simulink model "LRMate200Experimentor_Robot"  (R2015b)
settings: Solver=FixedStepDiscrete  StartTime=0.0  StopTime=10.0  FixedStep=si.SolverTimeStep  RelTol=1e-3
model workspace (MATLAB code in the model file):
  | rsi = evalin('base', 'si.ri{1}');
undefined symbols (not defined in the file or in its folder): si
libraries: simulink x4
(part 2 of 2)

== system LRMate200Experimentor_Robot/ModeSelection/Basic Control Mode/SwSrc9 ==
  S0 : Constant  Value=0
  S1 : Constant
  ST1 : Outport
  ST0 : Outport  Port=2
  wires:
  S0/1 -> ST0/1
  S1/1 -> ST1/1

== system LRMate200Experimentor_Robot/ModeSelection/LTT/SwSrc13 ==
  S0 : Constant  Value=0
  S1 : Constant
  ST1 : Outport
  ST0 : Outport  Port=2
  wires:
  S0/1 -> ST0/1
  S1/1 -> ST1/1

== system LRMate200Experimentor_Robot/ModeSelection/LTT/Triggered Subsystem ==
  In1 : Inport
  Trigger : TriggerPort  PortDimensions=1
  Data Store Write : DataStoreWrite  DataStoreName=ATI_ResidueOffset
  wires:
  In1/1 -> Data Store Write/1

== system LRMate200Experimentor_Robot/ModeSelection/LTT/Triggered Subsystem1 ==
  In1 : Inport
  Trigger : TriggerPort  TriggerType=falling
  Data Store Write1 : DataStoreWrite  DialogController=Simulink.DDGSource  DataStoreName=ATI_ResidueOffset
  wires:
  In1/1 -> Data Store Write1/1

== system LRMate200Experimentor_Robot/ModeSelection/Pos Run & Jog/Triggered Subsystem2 ==
  In1 : Inport
  Trigger : TriggerPort
  Data Store Write1 : DataStoreWrite  DialogController=Simulink.DDGSource  DataStoreName=RecordPosition
  wires:
  In1/1 -> Data Store Write1/1

== system LRMate200Experimentor_Robot/ModeSelection/Pos Run & Jog/Triggered Subsystem3 ==
  In1 : Inport
  Trigger : TriggerPort  TriggerType=falling
  Data Store Write1 : DataStoreWrite  DialogController=Simulink.DDGSource  DataStoreName=RecordPosition
  wires:
  In1/1 -> Data Store Write1/1

== system LRMate200Experimentor_Robot/PLAN_INTR_FLTR/Basic/double smoothing ==
  mcmd : Inport
  1st smoothing : Subsystem
  2nd smoothing : Subsystem
  alt_efot : Outport  InitialOutput=0
  wires:
  1st smoothing/1(out_1) -> 2nd smoothing/1(in_1)
  mcmd/1 -> 1st smoothing/1(in_1)
  2nd smoothing/1(out_1) -> alt_efot/1  "MotorVelCmd[2^20rev/itp]"

== system LRMate200Experimentor_Robot/ModeSelection/Basic Control Mode/ControllerMode/SafetyOverCheck ==
  Force_limit : Constant  Value=rsi.Force_limit
  PosOverCheck : MATLAB Function  TreatAsAtomicUnit=on  SystemSampleTime=si.itp
  Rate Transition{1..5} (5 alike) : RateTransition
  SafetyTrqLimit : Constant  Value=rsi.SafetyTrqLimit
  rj_pos_limit_max : Constant  Value=rsi.rj_pos_limit_max
  rj_pos_limit_min : Constant  Value=rsi.rj_pos_limit_min
  si.BASE_Z : Constant  Value=rsi.BASE_Z
  si.RADIUS : Constant  Value=rsi.RADIUS
  si.boundary_max : Constant  Value=rsi.boundary_max
  si.boundary_min : Constant  Value=rsi.boundary_min
  si.velboundary_max : Constant  Value=rsi.velboundary_max
  SafetyOver : Outport
  wires:
  rj_pos_limit_min/1 -> PosOverCheck/9(pos_limit_min)
  Rate Transition3/1 -> PosOverCheck/6(pos_deg)
  rj_pos_limit_max/1 -> PosOverCheck/10(pos_limit_max)
  [JointPos_deg] -> Rate Transition3/1  "RBJ_pos[deg]"
  PosOverCheck/1(SafetyOver) -> SafetyOver/1
  Rate Transition1/1 -> PosOverCheck/1(TransformationM)
  si.BASE_Z/1 -> PosOverCheck/2(BASE_Z)
  si.RADIUS/1 -> PosOverCheck/3(RADIUS)
  si.boundary_min/1 -> PosOverCheck/4(boundary_min)
  si.boundary_max/1 -> PosOverCheck/5(boundary_max)
  [TransformationM] -> Rate Transition1/1
  [JointVel_degs] -> Rate Transition2/1  "JointVel [deg/s]"
  Rate Transition2/1 -> PosOverCheck/7(jvel_degsec)
  si.velboundary_max/1 -> PosOverCheck/8(velboundary_max)
  [ATI_Force] -> Rate Transition4/1
  Force_limit/1 -> PosOverCheck/12(Force_Boundary)
  Rate Transition4/1 -> PosOverCheck/11(ATI_Force)
  [MotorTrqCmd_DSA] -> Rate Transition5/1  "MotorTrqCmd [DSA]"
  Rate Transition5/1 -> PosOverCheck/13(MotorTrqCmd_DSA)
  SafetyTrqLimit/1 -> PosOverCheck/14(MotorTrqCmd_DSA_Boundary)

== system LRMate200Experimentor_Robot/ModeSelection/Basic Control Mode/ControllerMode/SetTpPrgToMemory ==
  note: Use global variable si instead of model argument rsi because block parameters are not tunable
      | with model arguments (either workspace variable or simulink parameter object, either in scalar or structure)
  Trigger : TriggerPort  TriggerType=either
  Data Store Write : DataStoreWrite  DataStoreName=DS_ExtCmd_vcmd
  Data Store Write1 : DataStoreWrite  DialogController=Simulink.DDGSource  DataStoreName=DS_ExtCmd_vcmd_EndCnt
  Data Store Write2 : DataStoreWrite  DialogController=Simulink.DDGSource  DataStoreName=DS_ExtCmd_GripperCmd
  Data Store Write8 : DataStoreWrite  DialogController=Simulink.DDGSource  DataStoreName=DS_ExtCmd_inipos
  const_ExtCmd_grippercmd : Constant  Value=si.extcmd.grippercmd  VectorParams1D=off  SampleTime=-1
  const_ExtCmd_inipos : Constant  Value=si.extcmd.inipos_t  VectorParams1D=off  SampleTime=-1
  const_ExtCmd_vcmd : Constant  Value=si.extcmd.vcmd_t  SampleTime=-1
  const_ExtCmd_vcmd_EndCnt : Constant  Value=si.extcmd.vcmd_EndCnt_t  SampleTime=-1
  wires:
  const_ExtCmd_vcmd/1 -> Data Store Write/1
  const_ExtCmd_vcmd_EndCnt/1 -> Data Store Write1/1
  const_ExtCmd_inipos/1 -> Data Store Write8/1
  const_ExtCmd_grippercmd/1 -> Data Store Write2/1

== system LRMate200Experimentor_Robot/ModeSelection/Basic Control Mode/ControllerMode/Subsystem ==
  In1 : Inport
  Bitwise Operator : simulink/Logic and Bit Operations/Bitwise Operator  logicop=AND  UseBitMask=on  BitMask=bin2dec('000000001')  BitMaskRealWorld=Stored Integer
  Bitwise Operator1 : simulink/Logic and Bit Operations/Bitwise Operator  logicop=AND  UseBitMask=on  BitMask=bin2dec('10000000')  BitMaskRealWorld=Stored Integer
  Data Type Conversion : DataTypeConversion  OutDataTypeStr=boolean
  Data Type Conversion1 : DataTypeConversion  OutDataTypeStr=boolean
  Gain : Gain  Gain=1/2^7
  Rate Transition2 : RateTransition
  Out1 : Outport
  Out2 : Outport  Port=2
  wires:
  In1/1 -> Rate Transition2/1
  Bitwise Operator/1 -> Data Type Conversion/1
  Rate Transition2/1 -> Bitwise Operator1/1, Bitwise Operator/1
  Data Type Conversion/1 -> Out1/1
  Bitwise Operator1/1 -> Gain/1
  Data Type Conversion1/1 -> Out2/1
  Gain/1 -> Data Type Conversion1/1

== system LRMate200Experimentor_Robot/PLAN_INTR_FLTR/Basic/double smoothing/1st smoothing ==
  in_1 : Inport
  1/itp : Gain  Gain=1/(si.itp*1000)  SaturateOnIntegerOverflow=on  OutDataTypeStr=Inherit: Same as input  ParamDataTypeStr=Inherit: Same as input
  Delay{2..8,21} (8 alike) : UnitDelay  SampleTime=si.tsv
  Sum : Sum  Inputs=+++++++++  SaturateOnIntegerOverflow=on  InputSameDT=on  OutDataTypeStr=Inherit: Same as first input
  Sum1 : Sum  Inputs=+-  SaturateOnIntegerOverflow=on  InputSameDT=on  OutDataTypeStr=Inherit: Same as first input
  floor3 : Rounding
  itp : Gain  Gain=si.itp*1000  SaturateOnIntegerOverflow=on  OutDataTypeStr=Inherit: Same as input  ParamDataTypeStr=Inherit: Same as input
  out_1 : Outport  InitialOutput=0
  wires:
  floor3/1 -> itp/1, out_1/1
  1/itp/1 -> floor3/1
  itp/1 -> Sum1/2
  Sum/1 -> 1/itp/1, Sum1/1
  Sum1/1 -> Delay21/1
  Delay21/1 -> Sum/9
  Delay8/1 -> Sum/8
  Delay7/1 -> Sum/7, Delay8/1
  Delay6/1 -> Sum/6, Delay7/1
  Delay5/1 -> Sum/5, Delay6/1
  Delay4/1 -> Sum/4, Delay5/1
  Delay3/1 -> Sum/3, Delay4/1
  Delay2/1 -> Sum/2, Delay3/1
  in_1/1 -> Sum/1, Delay2/1

== system LRMate200Experimentor_Robot/PLAN_INTR_FLTR/Basic/double smoothing/2nd smoothing ==
  in_1 : Inport
  1/itp : Gain  Gain=1/(si.itp*1000)  SaturateOnIntegerOverflow=on  OutDataTypeStr=Inherit: Same as input  ParamDataTypeStr=Inherit: Same as input
  Delay{2..8,21} (8 alike) : UnitDelay  SampleTime=si.tsv
  Sum : Sum  Inputs=+++++++++  SaturateOnIntegerOverflow=on  InputSameDT=on  OutDataTypeStr=Inherit: Same as first input
  Sum1 : Sum  Inputs=+-  SaturateOnIntegerOverflow=on  InputSameDT=on  OutDataTypeStr=Inherit: Same as first input
  floor3 : Rounding
  itp : Gain  Gain=si.itp*1000  SaturateOnIntegerOverflow=on  OutDataTypeStr=Inherit: Same as input  ParamDataTypeStr=Inherit: Same as input
  out_1 : Outport  InitialOutput=0
  wires:
  floor3/1 -> out_1/1, itp/1
  Sum1/1 -> Delay21/1
  itp/1 -> Sum1/2
  1/itp/1 -> floor3/1
  Sum/1 -> 1/itp/1, Sum1/1
  Delay21/1 -> Sum/9
  Delay8/1 -> Sum/8
  in_1/1 -> Sum/1, Delay2/1
  Delay2/1 -> Sum/2, Delay3/1
  Delay3/1 -> Sum/3, Delay4/1
  Delay4/1 -> Sum/4, Delay5/1
  Delay5/1 -> Sum/5, Delay6/1
  Delay6/1 -> Sum/6, Delay7/1
  Delay7/1 -> Sum/7, Delay8/1

== matlab function LRMate200Experimentor_Robot/Measurement/Tilt Angle Esimation/MATLAB Function2 ==
  data: Button input; RecordData output; DATA input
function RecordData = Panel_RecordData(Button, DATA)

persistent Button_old  

if isempty(Button_old)
    Button_old = 0;
end

RecordData = zeros(size(DATA));
if Button > Button_old                %% press the button
        RecordData = DATA;     
end
    
Button_old = Button;

== stateflow chart LRMate200Experimentor_Robot/PLAN_INTR_FLTR/Basic/INTR ==
  settings: updateMethod=DISCRETE  sampleTime=si.itp
  state Mode [parallel]
    //movetime
    settings: executionOrder=1
    state Wait
      en: cnt=0;
      fdo=0;
    state Output
      en: cnt++;
      fdo=jvel_itp;
      out_ta1=ta1;
      out_ta2=ta2;
      du: cnt++;
    state HoldOutput
      en: fdo=0;
    (default) -> Wait
    Output -> Wait [order 3] : [VRDY==0]
    HoldOutput -> Wait
    Output -> Wait [order 1] : [cnt>=movetime_itp]
    Wait -> Output : [hasChanged(PlanDone_E)]
    Output -> HoldOutput [order 2] : [hasChanged(HoldPlanDo_E)]
  state Mode1 [parallel]
    // fltr_done_E
    settings: executionOrder=2
    state Wait1
      en: cnt_fltr=0;
    state during_output
      state Output1
        en: cnt_fltr++;
        du: cnt_fltr++;
      state HoldOutput1
        en: cnt_fltr=0;
        du: cnt_fltr++;
      Output1 -> HoldOutput1 [order 2] : [hasChanged(HoldPlanDo_E)]
    (default) -> Wait1
    during_output -> Wait1 : [VRDY==0]
        | {out_ta1=0; out_ta2=0; fltr_done_E;}
    HoldOutput1 -> Wait1 : [cnt_fltr>=ta1+ta2]
        | {out_ta1=0; out_ta2=0;}
        | / fltr_done_E
    Output1 -> Wait1 [order 1] : [cnt_fltr>=movetime_itp+ta1+ta2+1]
        | {out_ta1=0; out_ta2=0;}
        | / fltr_done_E
    Wait1 -> Output1 : [hasChanged(PlanDone_E)]
  data: jvel_itp input double size=[1 6]; fdo output double size=[1 6]; cnt local double size=1; movetime_itp input double size=1; ta1 input double size=1; ta2 input double size=1; PlanDone_E input boolean size=1; out_ta1 output double size=1; out_ta2 output double size=1; HoldPlanDo_E input boolean; cnt_fltr local double; VRDY input boolean
  events: fltr_done_E output EITHER_EDGE_EVENT

== stateflow chart LRMate200Experimentor_Robot/PLAN_INTR_FLTR/Basic/FLTR ==
  settings: updateMethod=DISCRETE  sampleTime=si.itp
  (default) -> (junction 57) : {do_reset=0;
      |  do_reset2=0;}
  (junction 57) -> (junction 65) [order 2]
  (junction 57) -> (junction 60) [order 1] : [hasChanged(fltr_done_E)]
      | {do_reset=1;}
  (junction 65) -> (junction 60)
  (junction 60) -> (junction 69) [order 2]
  (junction 60) -> (junction 68) [order 1] : [hasChanged(HoldSig_E)]
      | {do_reset2=1;}
  (junction 69) -> (junction 68)
  (junction 68) -> (junction 63) : {
      | vout3  = CalVcmd_2step_x(fdo_in,fta1,fta2,6,do_reset,do_reset2,va_s);
      |        // vout3 [ deg/itp ]
      |  vout_mpls =CalRbj2Mpls(vout3,k_rbj2mpls);
      |  out_vel=vout_mpls;
      |       // out_vel [ (2^20/rev)/itp ]
      | }
  data: vin function_input double size=[1 6]; flen1a function_input double size=1; flen2a function_input double size=1; AxisNum function_input double size=1; vout2 function_output double size=[1 6]; reset function_input double; reset2 function_input double; va function_input double size=[1 6]; mf_rbj function_input double size=[1 6]; mf_k_rbj2mpls function_input double size=[6 6]; mf_mpls function_output double size=[1 6]; fdo_in input double size=[1 6]; fta1 input double size=1; fta2 input double size=1; out_vel output double size=[1 6]; fltr_done_E input boolean; do_reset local double size=1; vout3 local double size=[1 6]; k_rbj2mpls input double size=[6 6] =rsi.k_rbj2mpls; vout_mpls local double size=[1 6]; va_s input double size=[1 6]; do_reset2 local double size=1; HoldSig_E input boolean size=1
  function vout2  = CalVcmd_2step_x(vin,flen1a,flen2a,AxisNum,reset,reset2,va):
    | function vout2  = CalVcmd_2step_x(vin,flen1a,flen2a,AxisNum,reset,reset2,va)
    | %CalVcmd1 
    | %
    | %
    | %vin 
    | %flen1a: 1
    | %flen2a:  2
    | %AxisNum: )
    | %reset: 1
    | %reset2: 1va
    | %va: rese2=1
    | %
    | %
    | %vout2: 
    | 
    | 
    | %
    | persistent f1 %
    | persistent ci1 %f
    | persistent f2 %
    | persistent ci2 %f
    | 
    | 
    | flen_max=500; %
    | flen1=flen1a+1; %flenflen0=1flen=2
    | flen2=flen2a+1; %flenflen0=1flen=2
    | 
    | %----------
    | if isempty(f1)
    |    f1 = zeros(flen_max,6);
    | end
    | if isempty(ci1)
    |    ci1 = 0;
    | end
    | if isempty(f2)
    |    f2 = zeros(flen_max,6);
    | end
    | if isempty(ci2)
    |    ci2 = 0;
    | end
    | 
    | %--------0------------
    | if reset==1
    |     ci1=0;
    |     ci2=0;
    |     
    |     %-----------------------------
    |     %0
    |     f1 = zeros(flen_max,6); 
    |     f2 = zeros(flen_max,6);
    |     %------------------------------
    | 
    | end
    | 
    | %--------va---------
    | if reset2==1
    |     ci1=0;
    |     ci2=0;
    |     
    |     %-----------------------------
    |     %va
    |     f1 = [ones(flen_max,1)*va(1,1) ...
    |           ones(flen_max,1)*va(1,2) ...
    |           ones(flen_max,1)*va(1,3) ...
    |           ones(flen_max,1)*va(1,4) ...
    |           ones(flen_max,1)*va(1,5) ...
    |           ones(flen_max,1)*va(1,6)]; 
    |       
    |       
    |     f2 = f1;
    |     %------------------------------
    | 
    | end
    | 
    | %---------1--------------
    | if ci1>=flen1
    |     ci1=0;
    | end
    | ci1=ci1+1;
    | f1(ci1,:)=vin;
    | 
    | %----------------------
    | %sum
    | %
    | vout1=sum(f1(1:flen1,:),1)/flen1;
    | %----------------------
    | 
    | %---------2--------------
    | if ci2>=flen2
    |     ci2=0;
    | end
    | ci2=ci2+1;
    | f2(ci2,:)=vout1;
    | 
    | %----------------------
    | %sum
    | %
    | vout2=sum(f2(1:flen2,:),1)/flen2;
    | %----------------------
    | 
    | end
  function mf_mpls  = CalRbj2Mpls(mf_rbj,mf_k_rbj2mpls):
    | function mf_mpls  = CalRbj2Mpls(mf_rbj,mf_k_rbj2mpls)
    | %CalRbj2Mpls 
    | %
    | %
    | %mf_rbj [deg] [1X6]
    | %       6J3J2
    | %      
    | %mf_k_rbj2mpls  
    | 
    | 
    | mf_mpls=(mf_k_rbj2mpls*mf_rbj')';
    | 
    | 
    | end

== stateflow chart LRMate200Experimentor_Robot/PLAN_INTR_FLTR/Basic/PLAN ==
  (default) -> (junction 10)
  (junction 10) -> (junction 25) [order 2] : [IniState == 1]
      | { [jpos_diff,jvel_s,jvel_itp_s,movetime_itp,ta1_s,ta2_s]=CalPlan ...
      |     (jvelmax_s,AccelTime1_s,AccelTime2_s,itp_s,AxisNum_s, ...
      |      pos1,pos3); }
  (junction 10) -> (junction 25) [order 1] : [IniState == 0]
      | { [jpos_diff,jvel_s,jvel_itp_s,movetime_itp,ta1_s,ta2_s]=CalPlan ...
      |     (jvelmax_s,AccelTime1_s,AccelTime2_s,itp_s,AxisNum_s, ...
      |      pos1,pos2); }
  (junction 25) -> (junction 38) : { PlanDone_E; }
  data: jvelmax function_input double size=[1 6]; AccelTime1 function_input double size=[1 6]; AccelTime2 function_input double size=[1 6]; itp function_input double size=1; AxisNum function_input double size=1; jpos1 function_input double size=[1 6]; jpos2 function_input double size=[1 6]; Pdiff function_output double size=[1 6]; jvel function_output double size=[1 6]; jvel_itp function_output double size=[1 6]; MoveTime function_output double size=1; taconsE1 function_output double size=1; taconsE2 function_output double size=1; ta1 temporary double size=[1 6]; ta2 temporary double size=[1 6]; pos1 input double size=6; jvelmax_s input double size=6 =si.jvelmax; AccelTime1_s input double size=6 =si.AccelTime1_s; AccelTime2_s input double size=6 =si.AccelTime2_s; itp_s local double size=1 =si.itp; AxisNum_s local double size=1 =si.AxisNum; jpos_diff output double size=6; jvel_s output double size=6; jvel_itp_s output double size=6; movetime_itp output double size=1; ta1_s output double size=1; ta2_s output double size=1; pos2 input double size=[1 6]; IniState input double; pos3 input double
  events: PlanDo_E input EITHER_EDGE_EVENT; PlanDone_E output EITHER_EDGE_EVENT
  function [Pdiff,jvel,jvel_itp,MoveTime,taconsE1,taconsE2] = CalPlan ...:
    | function [Pdiff,jvel,jvel_itp,MoveTime,taconsE1,taconsE2] = CalPlan ...
    |      ( jvelmax,AccelTime1,AccelTime2,itp,AxisNum,jpos1,jpos2)
    | %CalPlan PLAN
    | % 
    | %
    | %itp: itp[s]
    | %
    | %
    | %
    | %Pdiff: 1Ax
    | %jvel: 1Ax[deg/s]
    | %jvel_itp: 1Ax[deg/itp]
    | %MoveTime: MOVE_TIME[itp]
    | %taconsE1: 1[itp]
    | %taconsE2: 2[itp]
    | 
    | 
    | %
    | Pdiff=jpos2-jpos1;
    | Pdiff_abs=abs(Pdiff);
    | 
    | ta1=ceil((AccelTime1/1000)/itp); %1[itp]
    | ta2=ceil((AccelTime2/1000)/itp); %2[itp]
    | 
    | 
    | if all(Pdiff_abs==[0 0 0 0 0 0])
    |     %
    |     
    | %     jvel=zeros(1,AxisNum);  %zerosstateFlow
    |     jvel=[0 0 0 0 0 0];
    |     jvel_itp=[0 0 0 0 0 0];
    |     MoveTime=0;
    |     taconsE1=0;
    |     taconsE2=0;
    |  
    | else
    | 
    |     %
    |     %MoveTime0[s]
    |     [MoveTime0,maxMvtime_index]=max(Pdiff_abs./jvelmax);
    |     %MoveTime[itp]
    |     MoveTime=ceil(MoveTime0/itp);
    | 
    |     %
    |     jvel_itp=Pdiff/MoveTime;
    |     jvel=jvel_itp/itp;
    | 
    |     %
    |     ta_ratio=abs(jvel)./jvelmax;
    |     tacons1G=ceil(ta1.*ta_ratio);
    |     tacons2G=ceil(ta2.*ta_ratio);
    | 
    |     %
    |     [maxtacons,maxta_index]=max(tacons1G+tacons2G);
    |     taconsE1=tacons1G(maxta_index);
    |     taconsE2=tacons2G(maxta_index);
    |         %tacons1,tacons2ta_ratio
    |         %ta_ratio
    | end
    | 
    | end

== stateflow chart LRMate200Experimentor_Robot/PLAN_INTR_FLTR/JOG C/JOGC ==
  settings: updateMethod=DISCRETE  sampleTime=si.itp
  state Wait
    en: fdo=0;
  state Output_state
    state Output
      en:  fdo =JogC_CartesianVel(jog_axis_no,jog_speed_ratio,jog_direction);
      du:  fdo =JogC_CartesianVel(jog_axis_no,jog_speed_ratio,jog_direction);
    state HoldOutput
      en: fdo=0;
      cnt_fltr=0;
      du: cnt_fltr++;
    Output -> HoldOutput : [hasChanged(JogCCmd_E)]
  (default) -> Wait
  Output_state -> Wait : [VRDY==0]
      | / fltr_done_E_C
  (junction 114) -> Wait
  Wait -> Output : [hasChanged(JogCCmd_E)]
  HoldOutput -> (junction 114) : [cnt_fltr>=50]
      | / fltr_done_E_C
  data: jog_axis_no_in function_input double size=1; vel function_output double size=[1 6]; jog_speed_ratio_in function_input double size=1; jog_direction_in function_input double size=1; fdo output double size=[1 6]; cnt_fltr local double; VRDY input boolean; JogCCmd_E input boolean; jog_axis_no input double; jog_speed_ratio input double; jog_direction input double
  events: fltr_done_E_C output EITHER_EDGE_EVENT
  function vel  = JogC_CartesianVel(jog_axis_no_in,jog_speed_ratio_in,jog_direction_in):
    | function vel  = JogC_CartesianVel(jog_axis_no_in,jog_speed_ratio_in,jog_direction_in)
    | 
    | % Maximum Vel
    | Vmax = [0.1, 0.1, 0.1, 0.1745, 0.1745, 0.1745] ;    %   m/s         % rad/s
    | 
    | % Tool frame Velcoticy in Cartesian Space
    | vel = zeros(1,6);
    | vel(jog_axis_no_in)=Vmax(jog_axis_no_in)*(jog_speed_ratio_in/100)*jog_direction_in; %
    | 
    | end

== stateflow chart LRMate200Experimentor_Robot/PLAN_INTR_FLTR/Basic/Switch_VelCmdSource (MATLABchart) ==
  state ext_vel1
    en: cnt_itp=1;
    out_VelCmd=jogC_VelCmd';
    du: cnt_itp=cnt_itp+1;
    out_VelCmd= jogC_VelCmd';
  state ext_vel2
    en: cnt_itp=1;
    out_VelCmd=Force_VelCmd';
    du: cnt_itp=cnt_itp+1;
    out_VelCmd= Force_VelCmd';
  note: ext_vel(cnt_itp,:)
      | MATLAB
  state ini00_wait
  state ext_vel3
    en: cnt_itp=1;
    out_VelCmd=LTT_VelCmd';
    du: cnt_itp=cnt_itp+1;
    out_VelCmd= LTT_VelCmd';
  state inner_vel
    en: out_VelCmd=inner_VelCmd';
    du: out_VelCmd=inner_VelCmd';
  state ext_vel4
    en: cnt_itp=1;
    out_VelCmd=TI_VelCmd';
    du: cnt_itp=cnt_itp+1;
    out_VelCmd= TI_VelCmd';
  state ext_vel
    en: cnt_itp=1;
    out_VelCmd= ext_VelCmd';
    du: cnt_itp=cnt_itp+1;
    out_VelCmd= ext_VelCmd';
    %  ext_vel(cnt_itp,:)
    %  MATLAB
  state ext_vel_hold
    en: out_VelCmd=inner_VelCmd';
    du: out_VelCmd=inner_VelCmd';
  inner_vel -> ext_vel1 [order 5] : [hasChanged(JogCCmd_E)]
  (default) -> ini00_wait
  ext_vel1 -> inner_vel : [hasChanged(fltr_done_E_C)]
  inner_vel -> ext_vel2 [order 2] : [hasChanged(ForceCmd_E)]
  ext_vel2 -> inner_vel : [hasChanged(fltr_done_E_F)]
  ini00_wait -> inner_vel
  inner_vel -> ext_vel3 [order 4] : [hasChanged(LTTCmd_E)]
  ext_vel_hold -> inner_vel : [hasChanged(fltr_done_E)]
  ext_vel3 -> inner_vel : [hasChanged(fltr_done_E_L)]
  ext_vel -> inner_vel [order 2] : [hasChanged(fltr_done_E)]
  inner_vel -> ext_vel [order 1] : [hasChanged(ExtCmd_E)]
  ext_vel4 -> inner_vel : [hasChanged(fltr_done_E_TI)]
  inner_vel -> ext_vel4 [order 3] : [hasChanged(TICmd_E)]
  ext_vel -> ext_vel_hold [order 1] : [hasChanged(ExtCmd_Hold_E)]
  data: inner_VelCmd input double size=[1 6]; out_VelCmd output double size=6; cnt_itp local; ext_VelCmd input; ExtCmd_Hold_E input boolean size=1; fltr_done_E input boolean size=1; ExtCmd_E input boolean size=1; fltr_done_E_C input; JogCCmd_E input; jogC_VelCmd input; Force_VelCmd input; ForceCmd_E input; fltr_done_E_F input; fltr_done_E_L input; LTT_VelCmd input; LTTCmd_E input; fltr_done_E_TI input; TI_VelCmd input; TICmd_E input

== stateflow chart LRMate200Experimentor_Robot/PLAN_INTR_FLTR/Basic/FDO Source SW ==
  state CmdMode [parallel]
    settings: executionOrder=1
    state InnerCmd
      en,du:
      out_fdo=in1_fdo;
      out_ta1=in1_ta1;
      out_ta2=in1_ta2;
    state ReadyForCmd
      en:
      out_fdo=zero_fdo;
      out_ta1=0;
      out_ta2=0;
    state ExtCmd
      en,du:
      out_fdo=in2_fdo;
      out_ta1=in2_ta1;
      out_ta2=in2_ta2;
    state JogCmd
      en,du:
      out_fdo=in3_fdo;
      out_ta1=in3_ta1;
      out_ta2=in3_ta2;
    (default) -> (junction 76)
    (junction 74) -> (junction 76)
    (junction 76) -> ReadyForCmd
    (junction 65) -> (junction 74)
    ReadyForCmd -> InnerCmd [order 1] : [hasChanged(InnerCmd_E)]
    InnerCmd -> (junction 65) : fltr_done_E
    (junction 66) -> (junction 65)
    ReadyForCmd -> ExtCmd [order 2] : [hasChanged(ExtCmd_E)]
    ReadyForCmd -> JogCmd [order 3] : [hasChanged(JogCmd_E)]
    ExtCmd -> (junction 66) : fltr_done_E
    (junction 69) -> (junction 66)
    JogCmd -> (junction 69) : fltr_done_E
  state fltr_done_E_State [parallel]
    settings: executionOrder=2
    state fltr_done_E_Check
    (default) -> fltr_done_E_Check
    fltr_done_E_Check -> fltr_done_E_Check : [hasChanged(in1_fltr_done_E) |  hasChanged(in2_fltr_done_E) | hasChanged(in3_fltr_done_E)]
        | {out_fltr_done_E; }
        | / send(fltr_done_E,CmdMode);
  data: out_fdo output double size=[1 6]; out_ta1 output double; out_ta2 output double; in1_fdo input double size=[1 6]; in1_ta1 input double size=1; in1_ta2 input double size=1; in1_fltr_done_E input boolean; in2_fdo input double size=[1 6]; in2_ta1 input double size=1; in2_ta2 input double size=1; in2_fltr_done_E input boolean; in3_fdo input double size=[1 6]; in3_ta1 input double size=1; in3_ta2 input double size=1; in3_fltr_done_E input boolean; InnerCmd_E input boolean size=1; ExtCmd_E input boolean size=1; JogCmd_E input boolean size=1; zero_fdo constant double size=[1 6] =[0 0 0 0 0 0]
  events: out_fltr_done_E output EITHER_EDGE_EVENT; fltr_done_E local FUNCTION_CALL_EVENT

== stateflow chart LRMate200Experimentor_Robot/PLAN_INTR_FLTR/Basic/extcmd ==
  state ini00_wait
  state during_output
    state ext_vel
      en:
      out_VelCmd= DS_ExtCmd_vcmd(cnt_itp,:);
      out_GripperCmd= DS_ExtCmd_GripperCmd(cnt_itp,:);
      du:
      cnt_itp=cnt_itp+1;
      out_VelCmd= DS_ExtCmd_vcmd(cnt_itp,:);
      out_GripperCmd= DS_ExtCmd_GripperCmd(cnt_itp,:);
    state HoldDo
      en:
      out_vel_at_hold=out_VelCmd;
      out_VelCmd=[0 0 0 0 0 0];
      out_GripperCmd=[0 0 0 0 0 0];
      cnt_hold=0;
      du:
      cnt_hold = cnt_hold + 1;
    ext_vel -> HoldDo [order 1] : [hasChanged(ExtCmd_Hold_E)]
  (default) -> ini00_wait
  during_output -> ini00_wait : [VRDY==0]
      | {out_VelCmd=[0 0 0 0 0 0];
      | out_GripperCmd=[0 0 0 0 0 0];
      | fltr_done_E;}
  HoldDo -> ini00_wait : [cnt_hold>=hold_ta1+hold_ta2]
      | {fltr_done_E;}
  ext_vel -> ini00_wait [order 2] : [cnt_itp>= DS_ExtCmd_vcmd_EndCnt]
      | {out_VelCmd=[0 0 0 0 0 0];
      | out_GripperCmd=[0 0 0 0 0 0];
      | fltr_done_E;}
  ini00_wait -> ext_vel : [hasChanged(ExtCmd_E)]
      | {cnt_itp=1;}
  data: ExtCmd_E input boolean size=1; out_VelCmd output double size=[1 6]; cnt_itp local; DS_ExtCmd_vcmd data_store_memory; DS_ExtCmd_vcmd_EndCnt data_store_memory; ExtCmd_Hold_E input boolean size=1; out_vel_at_hold output size=[1 6]; hold_ta1 input; hold_ta2 input; cnt_hold local; VRDY input boolean; DS_ExtCmd_GripperCmd data_store_memory; out_GripperCmd output double size=[1 6]
  events: fltr_done_E output EITHER_EDGE_EVENT

== matlab function LRMate200Experimentor_Robot/Measurement/Force Sensor/Gravity Compensator ==
  data: W output; T input; PayloadG input; PayloadCG input
function W = gcomp(T,PayloadG,PayloadCG)
%#Gravity Compensation
R = T(1:3,1:3,6);   % Use the tool frame (J6 frame), which is the same as ATI frame
Fg = R'*PayloadG;
Tg = cross(PayloadCG,Fg);
W = [Fg; Tg];

== stateflow chart LRMate200Experimentor_Robot/PLAN_INTR_FLTR/JOG C/JOG1 ==
  settings: updateMethod=DISCRETE  sampleTime=si.itp
  state Wait
    en: fdo=0;
  state Output_state
    state Output
      en: [fdo,out_ta1,out_ta2] = CalJogAccTime ...
      (jog_jvelmax_s,AccelTime1_s,AccelTime2_s,itp_s, ...
      jog_axis_no_s,jog_speed_ratio_s,jog_direction_s);
    state HoldOutput
      en: fdo=0;
      cnt_fltr=0;
      du: cnt_fltr++;
    Output -> HoldOutput : [hasChanged(JogCCmd_E)]
  (default) -> Wait
  Output_state -> Wait : [VRDY==0]
      | {out_ta1=0; out_ta2=0;}
      | / fltr_done_E_C
  (junction 114) -> Wait
  Wait -> Output : [hasChanged(JogCCmd_E)]
  HoldOutput -> (junction 114) : [cnt_fltr>=out_ta1+out_ta2]
      | {out_ta1=0; out_ta2=0;}
      | / fltr_done_E_C
  data: jog_jvelmax function_input double size=[1 6]; AccelTime1 function_input double size=[1 6]; AccelTime2 function_input double size=[1 6]; itp function_input double size=1; jog_axis_no function_input double size=1; jvel_itp_vec function_output double size=[1 6]; ta1x function_output double size=1; ta2x function_output double size=1; ta1 temporary double size=1; ta2 temporary double size=1; jog_speed_ratio function_input double size=1; jog_direction function_input double size=1; fdo output double size=[1 6]; out_ta1 output double size=1; out_ta2 output double size=1; cnt_fltr local double; AccelTime1_s local double size=[1 6] =si.jog_AccelTime1_s; AccelTime2_s local double size=[1 6] =si.jog_AccelTime2_s; itp_s local double =si.itp; jog_jvelmax_s local double size=[1 6] =si.jog_jvelmax; jog_axis_no_s input double size=1; jog_speed_ratio_s input double size=1; jog_direction_s input double size=1; VRDY input boolean; JogCCmd_E input boolean
  events: fltr_done_E_C output EITHER_EDGE_EVENT
  function [jvel_itp_vec,ta1x,ta2x] = CalJogAccTime ...:
    | function [jvel_itp_vec,ta1x,ta2x] = CalJogAccTime ...
    |      (jog_jvelmax,AccelTime1,AccelTime2,itp,jog_axis_no,jog_speed_ratio,jog_direction)
    | %CalJogAccTime JOGFDO
    | % 
    | %
    | %jog_jvelmax: JOG[deg/s] 1Ax
    | %AccelTime1: JOG1[ms] 1Ax
    | %AccelTime2: JOG2[ms] 1Ax
    | %itp: itp[s]
    | %jog_axis_no: JOG(:16)
    | %jog_speed_ratio: JOG[%]
    | %jog_direction:JOG -1,0,1
    | %
    | %jvel_itp_vec: 1Ax[deg/itp]
    | %ta1x: 1[itp]
    | %ta2x: 2[itp]
    | 
    | ta1=ceil((AccelTime1(jog_axis_no)/1000)/itp); %1[itp] 
    | ta2=ceil((AccelTime2(jog_axis_no)/1000)/itp); %2[itp] 
    |     
    | %jog1itp[deg/itp]
    | jvel_itp_max=jog_jvelmax(jog_axis_no)*itp; %
    | %JOG[deg/itp]
    | jvel_itp=jvel_itp_max*(jog_speed_ratio/100)*jog_direction; %
    | 
    | %
    | jvel_itp_vec=zeros(1,6); %
    | jvel_itp_vec(jog_axis_no)=jvel_itp; %
    | 
    | %JOG
    | ta_ratio=abs(jvel_itp)/jvel_itp_max;
    | ta1x=ceil(ta1*ta_ratio);
    | ta2x=ceil(ta2*ta_ratio);
    | 
    | end

== stateflow chart LRMate200Experimentor_Robot/PLAN_INTR_FLTR/Basic/JOG ==
  settings: updateMethod=DISCRETE  sampleTime=si.itp
  state Wait
    en: fdo=0;
  state Output_state
    state Output
      en: [fdo,out_ta1,out_ta2] = CalJogAccTime ...
      (jog_jvelmax_s,AccelTime1_s,AccelTime2_s,itp_s, ...
      jog_axis_no_s,jog_speed_ratio_s,jog_direction_s);
    state HoldOutput
      en: fdo=0;
      cnt_fltr=0;
      du: cnt_fltr++;
    Output -> HoldOutput : [hasChanged(JogCmd_E)]
  (default) -> Wait
  Output_state -> Wait : [VRDY==0]
      | {out_ta1=0; out_ta2=0;}
      | / fltr_done_E
  (junction 114) -> Wait
  Wait -> Output : [hasChanged(JogCmd_E)]
  HoldOutput -> (junction 114) : [cnt_fltr>=out_ta1+out_ta2]
      | {out_ta1=0; out_ta2=0;}
      | / fltr_done_E
  data: jog_jvelmax function_input double size=[1 6]; AccelTime1 function_input double size=[1 6]; AccelTime2 function_input double size=[1 6]; itp function_input double size=1; jog_axis_no function_input double size=1; jvel_itp_vec function_output double size=[1 6]; ta1x function_output double size=1; ta2x function_output double size=1; ta1 temporary double size=1; ta2 temporary double size=1; jog_speed_ratio function_input double size=1; jog_direction function_input double size=1; fdo output double size=[1 6]; out_ta1 output double size=1; out_ta2 output double size=1; JogCmd_E input boolean; cnt_fltr local double; AccelTime1_s input double size=[1 6] =si.jog_AccelTime1_s; AccelTime2_s input double size=[1 6] =si.jog_AccelTime2_s; itp_s local double =si.itp; jog_jvelmax_s input double size=[1 6] =si.jog_jvelmax; jog_axis_no_s input double size=1; jog_speed_ratio_s input double size=1; jog_direction_s input double size=1; VRDY input boolean
  events: fltr_done_E output EITHER_EDGE_EVENT
  function [jvel_itp_vec,ta1x,ta2x] = CalJogAccTime ...:
    | function [jvel_itp_vec,ta1x,ta2x] = CalJogAccTime ...
    |      (jog_jvelmax,AccelTime1,AccelTime2,itp,jog_axis_no,jog_speed_ratio,jog_direction)
    | %CalJogAccTime JOGFDO
    | % 
    | %
    | %jog_jvelmax: JOG[deg/s] 1Ax
    | %AccelTime1: JOG1[ms] 1Ax
    | %AccelTime2: JOG2[ms] 1Ax
    | %itp: itp[s]
    | %jog_axis_no: JOG(:16)
    | %jog_speed_ratio: JOG[%]
    | %jog_direction:JOG -1,0,1
    | %
    | %jvel_itp_vec: 1Ax[deg/itp]
    | %ta1x: 1[itp]
    | %ta2x: 2[itp]
    | 
    | ta1=ceil((AccelTime1(jog_axis_no)/1000)/itp); %1[itp] 
    | ta2=ceil((AccelTime2(jog_axis_no)/1000)/itp); %2[itp] 
    |     
    | %jog1itp[deg/itp]
    | jvel_itp_max=jog_jvelmax(jog_axis_no)*itp; %
    | %JOG[deg/itp]
    | jvel_itp=jvel_itp_max*(jog_speed_ratio/100)*jog_direction; %
    | 
    | %
    | jvel_itp_vec=zeros(1,6); %
    | jvel_itp_vec(jog_axis_no)=jvel_itp; %
    | 
    | %JOG
    | ta_ratio=abs(jvel_itp)/jvel_itp_max;
    | ta1x=ceil(ta1*ta_ratio);
    | ta2x=ceil(ta2*ta_ratio);
    | 
    | end

== matlab function LRMate200Experimentor_Robot/PLAN_INTR_FLTR/Peg Hole Insertion/MATLAB Function ==
  data: VRDY input; ForceCmd_E input; JacobianT input; TCP_Force input; TCP_Pos input; Tilt_Angle input; JointVelCmd output; CartesianVelCmd output; fltr_done_E_F output; GMRpar_Priors input; GMRpar_Mu input; GMRpar_Sigma input; GMRpar_inv_SigmaIn input; GMRpar_det_SigmaIn input
function [JointVelCmd,CartesianVelCmd,fltr_done_E_F] = ForceControl_GMR(VRDY,ForceCmd_E,JacobianT,TCP_Force, TCP_Pos,Tilt_Angle, GMRpar_Priors ,GMRpar_Mu, GMRpar_Sigma, GMRpar_inv_SigmaIn,GMRpar_det_SigmaIn)

persistent fltr_done_E_F_old timeindex ForceCme_E_open

if isempty(fltr_done_E_F_old)
    fltr_done_E_F_old = false;
    timeindex = 0;
    ForceCme_E_open = false;
end

fltr_done_E_F = false;
JointVelCmd = zeros(1,6);
CartesianVelCmd = zeros(1,6);

if VRDY == 0     % system false
    fltr_done_E_F = ~fltr_done_E_F_old;
    JointVelCmd = zeros(1,6);
    ForceCme_E_open = false;
else     % VRDY == 1 system normal
    if ForceCmd_E == 1;        % turn on Force Control
        [JointVelCmd,CartesianVelCmd] = GMR_Force2qdot(JacobianT,TCP_Force, TCP_Pos, ForceCme_E_open ,Tilt_Angle, GMRpar_Priors ,GMRpar_Mu, GMRpar_Sigma, GMRpar_inv_SigmaIn,GMRpar_det_SigmaIn);
        ForceCme_E_open = true;
        %JointVelCmd = zeros(1,6);  
        
    else %ForceCmd_E == 0;   turn off Force Control
        JointVelCmd = zeros(1,6);
        if ForceCme_E_open == true;    % only if the Force Control has even been opened, then timestep begin to increase
            timeindex = timeindex + 1;
        end
        if timeindex > 50            % 50 timestep for smooth stop when Force Control turned off
            fltr_done_E_F = ~fltr_done_E_F_old;
            timeindex = 0 ;
            ForceCme_E_open = false;
        end
    end
end

%JointVelCmd = zeros(1,6);        %%% !!!!!!!!!!!!!!!

fltr_done_E_F_old = fltr_done_E_F;

== matlab function LRMate200Experimentor_Robot/PLAN_INTR_FLTR/JOG C/MATLAB Function1 ==
  data: Jacobian input; qdot output; vel input
function qdot = vel2qdot(Jacobian, vel)

q_dot = Jacobian\(vel');
qdot = q_dot';

== matlab function LRMate200Experimentor_Robot/PLAN_INTR_FLTR/LTT/MATLAB Function2 ==
  data: VRDY input; JointVelCmd output; LTTCmd_E input; LTT_ButtonE input; Jacobian input; LTT_Force input; fltr_done_E_L output; LTT_Gain input; LTT_Speed_Limit input
function [JointVelCmd, fltr_done_E_L] = ForceControl_LTT(VRDY, LTTCmd_E, LTT_ButtonE, Jacobian, LTT_Force, LTT_Gain, LTT_Speed_Limit)

persistent fltr_done_E_L_old

if isempty(fltr_done_E_L_old)
    fltr_done_E_L_old = false;
end

fltr_done_E_L = false;
JointVelCmd = zeros(1,6);

if VRDY == 0     % system false
    fltr_done_E_L = ~fltr_done_E_L_old;
    JointVelCmd = zeros(1,6); 
else     % VRDY == 1 system normal
    if (LTTCmd_E == 1) && (LTT_ButtonE == true) ;    % turn on Lead Through Teaching
        JointVelCmd = LTT_Force2qdot(Jacobian, LTT_Force, LTT_Gain, LTT_Speed_Limit);       
    elseif LTTCmd_E == 0            %LTTCmd_E == 0;   turn off Lead Through Teaching
        JointVelCmd = zeros(1,6);
        fltr_done_E_L = ~fltr_done_E_L_old;
    else
        JointVelCmd = zeros(1,6);
    end
end

fltr_done_E_L_old = fltr_done_E_L;

== matlab function LRMate200Experimentor_Robot/Measurement/LTT Handle/MATLAB Function ==
  data: LTT_Button input; LTTCmd_E input; RecordData output; DATA input; clock input; LTT_ButtonEnable output; RecordDataOn input; Record_Flag_Other input; Record_Flag_Self output
function [RecordData,  LTT_ButtonEnable, Record_Flag_Self] = LTT_RecordData(LTT_Button, LTTCmd_E, DATA, clock, RecordDataOn, Record_Flag_Other)

persistent LTT_Button_old  clock_click  GripperCmd_old

if isempty(LTT_Button_old)
    LTT_Button_old = 0;
    clock_click = 0;
    GripperCmd_old = zeros(6,1);
end

RecordData = zeros(size(DATA));

Record_Flag_Self = false;

if (RecordDataOn || Record_Flag_Other) && (clock - clock_click > 0.5)
    % (RecordDataOn used for Host PC controlled action). Do not record
    % data again within 0.5 sec (when RecordDataOn is reset)
    RecordData = DATA;
    %Record_Flag_Self = true;
    clock_click = clock;
end

if ~isequal(DATA(end-11:end-6), GripperCmd_old)    % if GripperCmd changes, also record data
    if clock > 2,  RecordData = DATA;  Record_Flag_Self = true;  end      % Record after application starts for 2 secs (initialization time)
    GripperCmd_old = DATA(end-11:end-6);
end

if LTTCmd_E     % LTT mode is enabled
    if LTT_Button > LTT_Button_old                  % press the button
        if (clock - clock_click < 1) && (clock - clock_click > 0.1)     % if double click, record data
            RecordData = DATA;
            Record_Flag_Self = true;
        end
        clock_click = clock;
    end
else
    GripperCmd_old = DATA(end-11:end-6);
end

LTT_ButtonEnable = false;
if LTT_Button == 1 && (clock - clock_click > 1)
    LTT_ButtonEnable = true;
end

LTT_Button_old = LTT_Button;

== matlab function LRMate200Experimentor_Robot/Measurement/Force Sensor/MATLAB Function6 ==
  data: ATI_Force input; TCP_Force output; L_ATI2TCP input; LTT_Force output; L_ATI2LTT input
function [TCP_Force, LTT_Force] = ForceTransform(ATI_Force, L_ATI2TCP, L_ATI2LTT)

% Add L_ATI2TCP and L_ATI2LTT as additional inputs and LTT_Force as additional output.
% -- Wenjie Chen, 2016/06/23

% ATI_Force: force/torque values at ATI sensor origin and sensor frame
% TCP_Force: force/torque values at TCP origin and robot tool frame
% LTT_Force: force/torque values at LTT handle grasping point and robot tool frame

% ATI frame and Tool frame have the same XYZ directions
TCP_Force = ATI_Force;
TCP_Force(4) = ATI_Force(4) + ATI_Force(2)*L_ATI2TCP(3) - ATI_Force(3)*L_ATI2TCP(2);
TCP_Force(5) = ATI_Force(5) - ATI_Force(1)*L_ATI2TCP(3) + ATI_Force(3)*L_ATI2TCP(1);
TCP_Force(6) = ATI_Force(6) + ATI_Force(1)*L_ATI2TCP(2) - ATI_Force(2)*L_ATI2TCP(1);

% ATI frame and Tool frame have the same XYZ directions
LTT_Force = ATI_Force;
LTT_Force(4) = ATI_Force(4) + ATI_Force(2)*L_ATI2LTT(3) - ATI_Force(3)*L_ATI2LTT(2);
LTT_Force(5) = ATI_Force(5) - ATI_Force(1)*L_ATI2LTT(3) + ATI_Force(3)*L_ATI2LTT(1);
LTT_Force(6) = ATI_Force(6) + ATI_Force(1)*L_ATI2LTT(2) - ATI_Force(2)*L_ATI2LTT(1);

== matlab function LRMate200Experimentor_Robot/Device Control/Gripper Input/MATLAB Function ==
  data: Green_Button input; Gripper_Mode output; Gripper_Drive output; clock input; Desired_Mode input
% Wenjie Chen, FANUC Corporation, 2016/06/29
% To control the gripper action by buttons. Here only two gripper modes are
% considered: 0-fully open and Desired_Mode. When double click the green
% button, the gripper mode is changed and executed.

function [Gripper_Mode, Gripper_Drive] = Gripper_Action(Green_Button, clock, Desired_Mode)

persistent Green_Button_old  Gripper_Mode_old  Gripper_Drive_old  clock_click

if isempty(Green_Button_old)
    Green_Button_old = 0;
    Gripper_Mode_old = 0;
    Gripper_Drive_old = false;
    clock_click = 0;
end

Gripper_Mode = Gripper_Mode_old;
if Gripper_Drive_old && (clock - clock_click < 0.032)   % if it is driving, make sure it should last at least 30ms
    Gripper_Drive = Gripper_Drive_old;
else
    Gripper_Drive = false;
end

if Green_Button ~= Green_Button_old                %% press the button
    if (clock - clock_click < 1) && (clock - clock_click > 0.1)      %% double click
        if Gripper_Mode_old
            Gripper_Mode = 0;
        else
            Gripper_Mode = Desired_Mode;
        end
        Gripper_Drive = true;
    end
    clock_click = clock;
end

Green_Button_old = Green_Button;
Gripper_Mode_old = Gripper_Mode;
Gripper_Drive_old = Gripper_Drive;

== matlab function LRMate200Experimentor_Robot/PLAN_INTR_FLTR/JOG C/MATLAB Function2 ==
  data: jogC_vel_cmd input; vel_cmd_C output; cur_tcp_pos input; boundary_min input; boundary_max input; Transformation_M input; T_B2W input
function vel_cmd_C = velC_cmd_adjust(jogC_vel_cmd, cur_tcp_pos, boundary_min, boundary_max, Transformation_M, T_B2W)

Rot_T2W = T_B2W(1:3,1:3) * Transformation_M(1:3,1:3,7);
vel_cmd_C_trans = Rot_T2W * jogC_vel_cmd(1:3);
slow_ratio = 0.3;
stop_zone = 0.01;
slow_zone = 0.05;

idx_out_limit = (cur_tcp_pos <= boundary_min + stop_zone * ones(3,1)) & vel_cmd_C_trans(1:3) < 0;
vel_cmd_C_trans(idx_out_limit) = 0;

idx_out_limit = (cur_tcp_pos >= boundary_max - stop_zone * ones(3,1)) & vel_cmd_C_trans(1:3) > 0;
vel_cmd_C_trans(idx_out_limit) = 0;

idx_out_limit = (cur_tcp_pos <= boundary_min + slow_zone * ones(3,1)) & vel_cmd_C_trans(1:3) < 0;
vel_cmd_C_trans(idx_out_limit) = vel_cmd_C_trans(idx_out_limit) * slow_ratio;

idx_out_limit = (cur_tcp_pos >= boundary_max - slow_zone * ones(3,1)) & vel_cmd_C_trans(1:3) > 0;
vel_cmd_C_trans(idx_out_limit) = vel_cmd_C_trans(idx_out_limit) * slow_ratio;

vel_cmd_C = [(Rot_T2W' * vel_cmd_C_trans); jogC_vel_cmd(4:6)];

== matlab function LRMate200Experimentor_Robot/PLAN_INTR_FLTR/Peg Hole Insertion/MATLAB Function3 ==
  data: VRDY input; JointVelCmd output; TICmd_E input; JacobianT input; TCP_Force input; fltr_done_E_TI output
function [JointVelCmd,fltr_done_E_TI] = ForceControl_TI(VRDY,TICmd_E, JacobianT,TCP_Force)

persistent fltr_done_E_TI_old

if isempty(fltr_done_E_TI_old)
    fltr_done_E_TI_old = false;
end

fltr_done_E_TI = false;
JointVelCmd = zeros(1,6);

if VRDY == 0     % system false
    fltr_done_E_TI = ~fltr_done_E_TI_old;
    JointVelCmd = zeros(1,6); 
else     % VRDY == 1 system normal
    if (TICmd_E == 1)    % turn on Lead Through Teaching
        JointVelCmd = TiltIn_Force2qdot(JacobianT,TCP_Force);       
    elseif TICmd_E == 0            %LTTCmd_E == 0;   turn off Lead Through Teaching
        JointVelCmd = zeros(1,6);
        fltr_done_E_TI = ~fltr_done_E_TI_old;
    else
        JointVelCmd = zeros(1,6);
    end
end

fltr_done_E_TI_old = fltr_done_E_TI;

== matlab function LRMate200Experimentor_Robot/Measurement/Tilt Angle Esimation/TiltEstimate ==
  data: TCP_Force input; TiltANA_col output; TransformationM input; Alpha output; JointPos_deg input
function [TiltANA_col,Alpha] = TiltEstimation(TCP_Force, TransformationM, JointPos_deg ) 

Fx = TCP_Force(1);
Fz = -TCP_Force(3);
My = -TCP_Force(5);

%L = 0.08 + 0.196 + 0.062; % distance from wrist to peg end

% Px = TCP_Pos(1);
% Py = TCP_Pos(2);
% Pz = TCP_Pos(3);

r = 25.369/2/1000;   % m  !!!!!!!!!!!!!!!! wrong! /2

Estimate1 = atand((sqrt(4*r^2*Fx^2+4*r*Fz*My) - 2*r*Fx) / (2*r*Fz))*2;
% at FANUC
%Alpha = Estimate1*0.9206-19;   % (deg) line compensate from test data    17.8644
% at Berkeley
Alpha = Estimate1*1.3164-13.01;   % (deg) line compensate from test data

TiltANA_col = [reshape(TransformationM(:,:,7),16,1);JointPos_deg; Alpha];

% 
% deltaX = r*(1-cosd(Alpha));
% deltaY = 0;    %% what if hole is not in the x axis
% deltaZ = r*(1-cosd(Alpha))/(1+cosd(Alpha))*sind(Alpha) ;    % 1cm above the hole ;
% 
% 

%% 
% Theta_Base2Hole = TiltAngle - Alpha;
% R_Base2Hole = [ cosd(-Theta_Base2Hole),   0,   sind(-Theta_Base2Hole) ;
%                           0,              1,   0           ;
%                -sind(-Theta_Base2Hole),   0,   cosd(-Theta_Base2Hole)];
% P_peg_new =  TransformationM(1:3,4,7) + R_Base2Hole*[-deltaX ; 0 ; -deltaZ + 0.01 ];
% 
% P_3_new = P_peg_new + [-L*sind(Theta_Base2Hole); 0; L*cosd(Theta_Base2Hole)];
% 
% JointPosNew_deg = zeros(6,1);

== matlab function LRMate200Experimentor_Robot/PLAN_INTR_FLTR/JOG C/MATLAB Function3 ==
  data: jogJ_vel_cmd input; vel_cmd_J output; cur_jnt_pos input; boundary_min input; boundary_max input
function vel_cmd_J = velJ_cmd_adjust(jogJ_vel_cmd, cur_jnt_pos, boundary_min, boundary_max)

vel_cmd_J = jogJ_vel_cmd;
slow_ratio = 0.3;
stop_zone = 2;
slow_zone = 10;

idx_out_limit = (cur_jnt_pos <= boundary_min + stop_zone * ones(6,1)) & vel_cmd_J(:) < 0;
vel_cmd_J(idx_out_limit) = 0;

idx_out_limit = (cur_jnt_pos >= boundary_max - stop_zone * ones(6,1)) & vel_cmd_J(:) > 0;
vel_cmd_J(idx_out_limit) = 0;

idx_out_limit = (cur_jnt_pos <= boundary_min + slow_zone * ones(6,1)) & vel_cmd_J(:) < 0;
vel_cmd_J(idx_out_limit) = vel_cmd_J(idx_out_limit) * slow_ratio;

idx_out_limit = (cur_jnt_pos >= boundary_max - slow_zone * ones(6,1)) & vel_cmd_J(:) > 0;
vel_cmd_J(idx_out_limit) = vel_cmd_J(idx_out_limit) * slow_ratio;

== matlab function LRMate200Experimentor_Robot/ModeSelection/Basic Control Mode/ControllerMode/SafetyOverCheck/PosOverCheck ==
  data: TransformationM input; BASE_Z input; RADIUS input; boundary_min input; boundary_max input; pos_deg input; jvel_degsec input; velboundary_max input; SafetyOver output; pos_limit_min input; pos_limit_max input; ATI_Force input; Force_Boundary input; MotorTrqCmd_DSA input; MotorTrqCmd_DSA_Boundary input
function SafetyOver = SafetyOverCheck ...
     (TransformationM, BASE_Z, RADIUS, boundary_min, boundary_max, pos_deg, jvel_degsec, ...
     velboundary_max, pos_limit_min, pos_limit_max, ATI_Force, Force_Boundary, MotorTrqCmd_DSA, MotorTrqCmd_DSA_Boundary)

if any((pos_deg < pos_limit_min) | (pos_deg > pos_limit_max))  
    SafetyOver = 1;   % Position Over
elseif any(abs(jvel_degsec) > velboundary_max)
    SafetyOver = 2;   % Velocity Over 
elseif any(abs(ATI_Force) > Force_Boundary)
    SafetyOver = 3;   % Force Over 
elseif any(abs(MotorTrqCmd_DSA) > MotorTrqCmd_DSA_Boundary)
    SafetyOver = 4;   % Motor Torque Cmd Over 
else
    SafetyOver = safety_check(TransformationM, BASE_Z, RADIUS, boundary_min, boundary_max);  % Boundary & Self Collision 
end

== matlab function LRMate200Experimentor_Robot/PLAN_INTR_FLTR/LTT/MATLAB Function4 ==
  data: VRDY input; JointVelCmd output size=[1,6]; RepFCmd_E input; LTT_ButtonE input; Jacobian input; DoF input; Repulsive_Force input; RepF_Gain input; CartVelCmd output
function [JointVelCmd, CartVelCmd]  = ForceControl_RepF(VRDY,RepFCmd_E, LTT_ButtonE, Jacobian, DoF, Repulsive_Force,RepF_Gain)

CartVelCmd = zeros(1,6);
JointVelCmd = zeros(1,6);

if VRDY == 0     % system false
    JointVelCmd = zeros(1,6);
    CartVelCmd = zeros(1,6);
    
else     % VRDY == 1 system normal
    if (RepFCmd_E == 1) %&& (LTT_ButtonE == true);    % turn on Lead Through Teaching
        [JointVelCmd, CartVelCmd] = RepF_Force2qdot(Jacobian,Repulsive_Force, DoF, RepF_Gain);       
    elseif RepFCmd_E == 0            %LTTCmd_E == 0;   turn off Lead Through Teaching
        JointVelCmd = zeros(1,6);
        CartVelCmd = zeros(1,6);
    else
        JointVelCmd = zeros(1,6);
         CartVelCmd = zeros(1,6);
    end
end
